simulink model "GSM_sim_orig"  (Simulink 8.1)
settings: Solver=VariableStepDiscrete  StartTime=0.0  StopTime=simulationTime  RelTol=1e-3
undefined symbols (not defined in the file): get, lengthOfSymbol, sampleTime
libraries: commsink2 x9, commchan3 x3, commdigbbndcpm2 x2, commdigbbndpm3 x1, commutil2 x1, dspsigops x1
settings Model: Creator=Philipp Fetzer  LastModifiedBy=mainster
settings OptimizationCC: ExpressionDepthLimit=128
settings DebuggingCC: StrictBusMsg=Warning

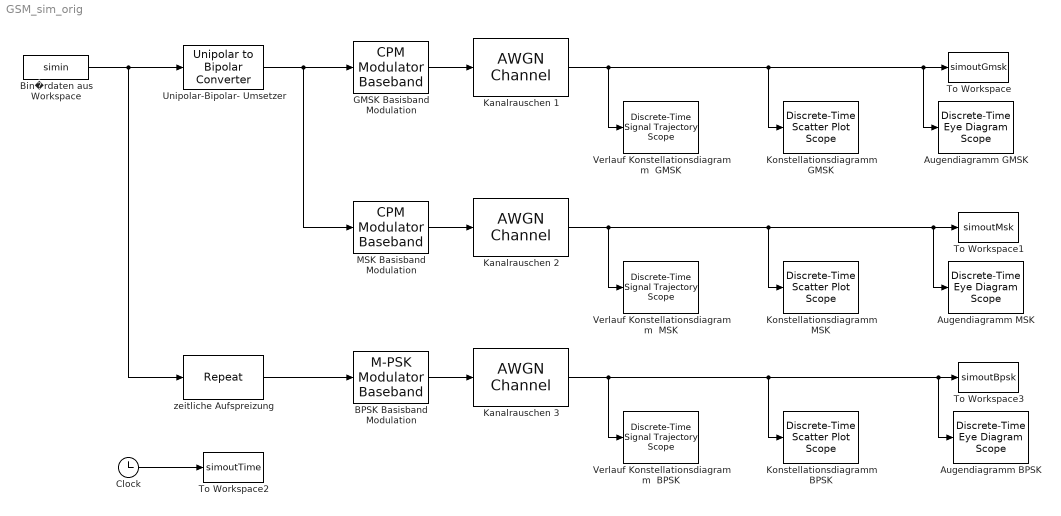
== system GSM_sim_orig ==
  Augendiagramm BPSK : commsink2/Discrete-Time Eye Diagram Scope  Tag=EyeDiagram  sampPerSymb=lengthOfSymbol  offsetEye=0  symbPerTrace=2  numTraces=40  numNewFrames=10  LineStyles=-  LineColors=b  dupPoints=on  fading=on  render=on  AxisGrid=on  yMin=-1.5  yMax=1.5  inphaseLabel=Amplitude Realteil  quadratureLabel=Amplitude Imaginaerteil  openScopeAtSimStart=on  dispDiagram=In-phase and Quadrature  FrameNumber=off  FigPos=get(0,'defaultfigureposition');  figTitle=Augendiagramm (2 Symbole)  block_type_=eye  numLinesMax=8
  Augendiagramm GMSK : commsink2/Discrete-Time Eye Diagram Scope  Tag=EyeDiagram  sampPerSymb=lengthOfSymbol  offsetEye=0  symbPerTrace=2  numTraces=80  numNewFrames=10  LineStyles=-  LineColors=b  dupPoints=on  fading=on  render=on  AxisGrid=on  yMin=-1.5  yMax=1.5  inphaseLabel=Amplitude Realteil  quadratureLabel=Amplitude Imaginaerteil  openScopeAtSimStart=on  dispDiagram=In-phase and Quadrature  FrameNumber=off  FigPos=get(0,'defaultfigureposition');  figTitle=Augendiagramm (2 Symbole)  block_type_=eye  numLinesMax=8
  "Augendiagramm MSK " : commsink2/Discrete-Time Eye Diagram Scope  Tag=EyeDiagram  sampPerSymb=lengthOfSymbol  offsetEye=0  symbPerTrace=2  numTraces=40  numNewFrames=10  LineStyles=-  LineColors=b  dupPoints=on  fading=on  render=on  AxisGrid=on  yMin=-1.5  yMax=1.5  inphaseLabel=Amplitude Realteil  quadratureLabel=Amplitude Imaginaerteil  openScopeAtSimStart=on  dispDiagram=In-phase and Quadrature  FrameNumber=off  FigPos=get(0,'defaultfigureposition');  figTitle=Augendiagramm (2 Symbole)  block_type_=eye  numLinesMax=8
  BPSK Basisband Modulation : commdigbbndpm3/M-PSK Modulator Baseband  M=2  InType=Integer  Enc=Binary  Mapping=[0:2]  Ph=phaseOffset  outDtype=double  outWordLen=16  outUDDataType=sfix(16)  outFracLenMode=Best precision  outFracLen=15
  Bin�rdaten aus Workspace : FromWorkspace  VariableName=simin  SampleTime=sampleTime
  Clock : Clock
  GMSK Basisband Modulation : commdigbbndcpm2/CPM Modulator Baseband  Mnum=2  inputType=Integer  mappingType=Binary  modIdx=.5  pulseShape=Gaussian  BT=.3  mainLobePulseLength=0.2  rollOff=0.2  pulseLength=4  preHistory=1  phaseOffset=phaseOffset  samplesPerSymbol=lengthOfSymbol  RateOptions=Inherit from input (this choice will be removed - see release notes)  outDataType=double
  Kanalrauschen 1 : commchan3/AWGN Channel  InputProcessing=Inherited (this choice will be removed - see release notes)  seed=67  noiseMode="Signal to noise ratio  (SNR)"  EbNodB=30  EsNodB=10  SNRdB=SNR  bitsPerSym=1  Ps=1  Tsym=1  variance=1
  Kanalrauschen 2 : commchan3/AWGN Channel  InputProcessing=Inherited (this choice will be removed - see release notes)  seed=67  noiseMode="Signal to noise ratio  (SNR)"  EbNodB=30  EsNodB=10  SNRdB=SNR  bitsPerSym=1  Ps=1  Tsym=1  variance=1
  Kanalrauschen 3 : commchan3/AWGN Channel  InputProcessing=Inherited (this choice will be removed - see release notes)  seed=67  noiseMode="Signal to noise ratio  (SNR)"  EbNodB=30  EsNodB=10  SNRdB=SNR  bitsPerSym=1  Ps=1  Tsym=1  variance=1
  Konstellationsdiagramm BPSK : commsink2/Discrete-Time Scatter Plot Scope  Tag=ScatterPlot  sampPerSymb=lengthOfSymbol  offsetEye=0  numTraces=150  numNewFrames=20  LineMarkers=.  LineColors=b  fading=on  render=on  AxisGrid=on  xMin=-1.3  xMax=1.315  yMin=-1.3  yMax=1.315  inphaseLabel=Amplitude Realteil  quadratureLabel=Amplitude Imaginaerteil  openScopeAtSimStart=on  FrameNumber=off  FigPos=[414 218 560 420]  figTitle=Konstellationsdiagramm  numLinesMax=8  block_type_=scatter
  Konstellationsdiagramm GMSK : commsink2/Discrete-Time Scatter Plot Scope  Tag=ScatterPlot  sampPerSymb=lengthOfSymbol  offsetEye=0  numTraces=150  numNewFrames=20  LineMarkers=.  LineColors=b  fading=on  render=on  AxisGrid=on  xMin=-1.3  xMax=1.315  yMin=-1.3  yMax=1.315  inphaseLabel=Amplitude Realteil  quadratureLabel=Amplitude Imaginaerteil  openScopeAtSimStart=on  FrameNumber=off  FigPos=get(0,'defaultfigureposition');  figTitle=Konstellationsdiagramm  numLinesMax=8  block_type_=scatter
  "Konstellationsdiagramm MSK " : commsink2/Discrete-Time Scatter Plot Scope  Tag=ScatterPlot  sampPerSymb=lengthOfSymbol  offsetEye=0  numTraces=150  numNewFrames=20  LineMarkers=.  LineColors=b  fading=on  render=on  AxisGrid=on  xMin=-1.3  xMax=1.315  yMin=-1.3  yMax=1.315  inphaseLabel=Amplitude Realteil  quadratureLabel=Amplitude Imaginaerteil  openScopeAtSimStart=on  FrameNumber=off  FigPos=get(0,'defaultfigureposition');  figTitle=Konstellationsdiagramm  numLinesMax=8  block_type_=scatter
  MSK Basisband Modulation : commdigbbndcpm2/CPM Modulator Baseband  Mnum=2  inputType=Integer  mappingType=Binary  modIdx=0.5  pulseShape=Rectangular  BT=0.3  mainLobePulseLength=0.2  rollOff=0.2  pulseLength=1  preHistory=1  phaseOffset=phaseOffset  samplesPerSymbol=lengthOfSymbol  RateOptions=Inherit from input (this choice will be removed - see release notes)  outDataType=double
  To Workspace : ToWorkspace  VariableName=simoutGmsk  SampleTime=-1  SaveFormat=Structure
  To Workspace1 : ToWorkspace  VariableName=simoutMsk  SampleTime=-1  SaveFormat=Structure
  To Workspace2 : ToWorkspace  VariableName=simoutTime  SampleTime=-1  SaveFormat=Structure
  To Workspace3 : ToWorkspace  VariableName=simoutBpsk  SampleTime=-1  SaveFormat=Structure
  Unipolar-Bipolar- Umsetzer : commutil2/Unipolar to Bipolar Converter  M=2  polarity=Positive  dataType=Inherit via internal rule
  Verlauf Konstellationsdiagramm  BPSK : commsink2/Discrete-Time Signal Trajectory Scope  Tag=SignalTrajectory  sampPerSymb=lengthOfSymbol  offsetEye=0  numTraces=40  numNewFrames=10  LineStyles=-  LineColors=b  fading=on  render=on  AxisGrid=on  xMin=-1.05  xMax=1.05  yMin=-1.05  yMax=1.05  inphaseLabel=Amplitude Realteil  quadratureLabel=Amplitude Imaginaerteil  openScopeAtSimStart=on  FrameNumber=off  FigPos=get(0,'defaultfigureposition');  figTitle=Verlauf Konstellationsdiagramm  numLinesMax=8  block_type_=xy
  Verlauf Konstellationsdiagramm  GMSK : commsink2/Discrete-Time Signal Trajectory Scope  Tag=SignalTrajectory  sampPerSymb=lengthOfSymbol  offsetEye=0  numTraces=40  numNewFrames=10  LineStyles=-  LineColors=b  fading=on  render=on  AxisGrid=on  xMin=-1.3  xMax=1.315  yMin=-1.3  yMax=1.315  inphaseLabel=Amplitude Realteil  quadratureLabel=Amplitude Imaginaerteil  openScopeAtSimStart=on  FrameNumber=off  FigPos=get(0,'defaultfigureposition');  figTitle=Verlauf Konstellationsdiagramm  numLinesMax=8  block_type_=xy
  "Verlauf Konstellationsdiagramm  MSK " : commsink2/Discrete-Time Signal Trajectory Scope  Tag=SignalTrajectory  sampPerSymb=lengthOfSymbol  offsetEye=0  numTraces=40  numNewFrames=10  LineStyles=-  LineColors=b  fading=on  render=on  AxisGrid=on  xMin=-1.3  xMax=1.315  yMin=-1.3  yMax=1.315  inphaseLabel=Amplitude Realteil  quadratureLabel=Amplitude Imaginaerteil  openScopeAtSimStart=on  FrameNumber=on  FigPos=[2548 512 560 420]  figTitle=Verlauf Konstellationsdiagramm  numLinesMax=8  block_type_=xy
  zeitliche Aufspreizung : dspsigops/Repeat  N=lengthOfSymbol  InputProcessing=Inherited (this choice will be removed - see release notes)  RateOptions=Allow multirate processing  ic=0  mode=Unused parameter value
  wires:
  Unipolar-Bipolar- Umsetzer/1 -> GMSK Basisband Modulation/1, MSK Basisband Modulation/1
  MSK Basisband Modulation/1 -> Kanalrauschen 2/1
  Bin�rdaten aus Workspace/1 -> Unipolar-Bipolar- Umsetzer/1, zeitliche Aufspreizung/1
  Clock/1 -> To Workspace2/1
  Kanalrauschen 1/1 -> Augendiagramm GMSK/1, To Workspace/1, Konstellationsdiagramm GMSK/1, Verlauf Konstellationsdiagramm  GMSK/1
  GMSK Basisband Modulation/1 -> Kanalrauschen 1/1
  zeitliche Aufspreizung/1 -> BPSK Basisband Modulation/1
  BPSK Basisband Modulation/1 -> Kanalrauschen 3/1
  Kanalrauschen 2/1 -> "Verlauf Konstellationsdiagramm  MSK "/1, To Workspace1/1, "Augendiagramm MSK "/1, "Konstellationsdiagramm MSK "/1
  Kanalrauschen 3/1 -> To Workspace3/1, Augendiagramm BPSK/1, Konstellationsdiagramm BPSK/1, Verlauf Konstellationsdiagramm  BPSK/1
